simulink model "ALL_Test"  (R2021b)
settings: Solver=VariableStepAuto  StartTime=0.0  StopTime=0.1  RelTol=1e-3
undefined symbols (not defined in the file): ac, ma
libraries: fl_lib x142, nesl_utility x5, sdl_lib x1
settings Model: Creator=김웅지  LastModifiedBy=김웅지

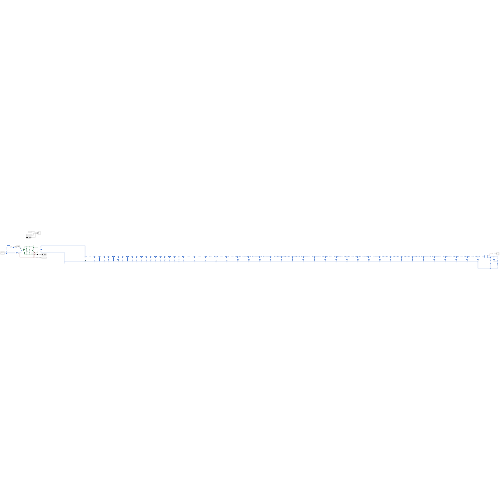
[thumbnail: Simulink's stored preview of the top-level diagram]
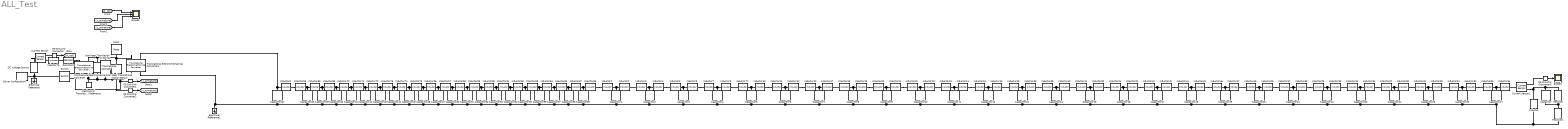
== system ALL_Test ==
  Capacitor : fl_lib/Electrical/Electrical Elements/Capacitor  c=ac.rad.Cm1 F  r=1e-15 Ohm  g=0 1/Ohm  i_specify=off  i_priority=None  i=0 A  i_nominal_specify=off  i_nominal_unit=A  i_nominal_value=1  v_specify=off  v_priority=None  v=0 V  v_nominal_specify=off  v_nominal_unit=V  v_nominal_value=1  vc_specify=off  vc_priority=High  vc=0 V  vc_nominal_specify=off  vc_nominal_unit=V  vc_nominal_value=1
  Capacitor1 : fl_lib/Electrical/Electrical Elements/Capacitor  c=ac.ho.C(1) F  r=1e-15 Ohm  g=0 1/Ohm  i_specify=off  i_priority=None  i=0 A  i_nominal_specify=off  i_nominal_unit=A  i_nominal_value=1  v_specify=off  v_priority=None  v=0 V  v_nominal_specify=off  v_nominal_unit=V  v_nominal_value=1  vc_specify=off  vc_priority=High  vc=0 V  vc_nominal_specify=off  vc_nominal_unit=V  vc_nominal_value=1
  Capacitor10 : fl_lib/Electrical/Electrical Elements/Capacitor  c=ac.ho.C(10) F  r=1e-15 Ohm  g=0 1/Ohm  i_specify=off  i_priority=None  i=0 A  i_nominal_specify=off  i_nominal_unit=A  i_nominal_value=1  v_specify=off  v_priority=None  v=0 V  v_nominal_specify=off  v_nominal_unit=V  v_nominal_value=1  vc_specify=off  vc_priority=High  vc=0 V  vc_nominal_specify=off  vc_nominal_unit=V  vc_nominal_value=1
  Capacitor11 : fl_lib/Electrical/Electrical Elements/Capacitor  c=ac.ho.C(11) F  r=1e-15 Ohm  g=0 1/Ohm  i_specify=off  i_priority=None  i=0 A  i_nominal_specify=off  i_nominal_unit=A  i_nominal_value=1  v_specify=off  v_priority=None  v=0 V  v_nominal_specify=off  v_nominal_unit=V  v_nominal_value=1  vc_specify=off  vc_priority=High  vc=0 V  vc_nominal_specify=off  vc_nominal_unit=V  vc_nominal_value=1
  Capacitor12 : fl_lib/Electrical/Electrical Elements/Capacitor  c=ac.ho.C(12) F  r=1e-15 Ohm  g=0 1/Ohm  i_specify=off  i_priority=None  i=0 A  i_nominal_specify=off  i_nominal_unit=A  i_nominal_value=1  v_specify=off  v_priority=None  v=0 V  v_nominal_specify=off  v_nominal_unit=V  v_nominal_value=1  vc_specify=off  vc_priority=High  vc=0 V  vc_nominal_specify=off  vc_nominal_unit=V  vc_nominal_value=1
  Capacitor13 : fl_lib/Electrical/Electrical Elements/Capacitor  c=ac.ho.C(13) F  r=1e-15 Ohm  g=0 1/Ohm  i_specify=off  i_priority=None  i=0 A  i_nominal_specify=off  i_nominal_unit=A  i_nominal_value=1  v_specify=off  v_priority=None  v=0 V  v_nominal_specify=off  v_nominal_unit=V  v_nominal_value=1  vc_specify=off  vc_priority=High  vc=0 V  vc_nominal_specify=off  vc_nominal_unit=V  vc_nominal_value=1
  Capacitor14 : fl_lib/Electrical/Electrical Elements/Capacitor  c=ac.ho.C(14) F  r=1e-15 Ohm  g=0 1/Ohm  i_specify=off  i_priority=None  i=0 A  i_nominal_specify=off  i_nominal_unit=A  i_nominal_value=1  v_specify=off  v_priority=None  v=0 V  v_nominal_specify=off  v_nominal_unit=V  v_nominal_value=1  vc_specify=off  vc_priority=High  vc=0 V  vc_nominal_specify=off  vc_nominal_unit=V  vc_nominal_value=1
  Capacitor15 : fl_lib/Electrical/Electrical Elements/Capacitor  c=ac.ho.C(15) F  r=1e-15 Ohm  g=0 1/Ohm  i_specify=off  i_priority=None  i=0 A  i_nominal_specify=off  i_nominal_unit=A  i_nominal_value=1  v_specify=off  v_priority=None  v=0 V  v_nominal_specify=off  v_nominal_unit=V  v_nominal_value=1  vc_specify=off  vc_priority=High  vc=0 V  vc_nominal_specify=off  vc_nominal_unit=V  vc_nominal_value=1
  Capacitor16 : fl_lib/Electrical/Electrical Elements/Capacitor  c=ac.ho.C(16) F  r=1e-15 Ohm  g=0 1/Ohm  i_specify=off  i_priority=None  i=0 A  i_nominal_specify=off  i_nominal_unit=A  i_nominal_value=1  v_specify=off  v_priority=None  v=0 V  v_nominal_specify=off  v_nominal_unit=V  v_nominal_value=1  vc_specify=off  vc_priority=High  vc=0 V  vc_nominal_specify=off  vc_nominal_unit=V  vc_nominal_value=1
  Capacitor17 : fl_lib/Electrical/Electrical Elements/Capacitor  c=ac.ho.C(17) F  r=1e-15 Ohm  g=0 1/Ohm  i_specify=off  i_priority=None  i=0 A  i_nominal_specify=off  i_nominal_unit=A  i_nominal_value=1  v_specify=off  v_priority=None  v=0 V  v_nominal_specify=off  v_nominal_unit=V  v_nominal_value=1  vc_specify=off  vc_priority=High  vc=0 V  vc_nominal_specify=off  vc_nominal_unit=V  vc_nominal_value=1
  Capacitor18 : fl_lib/Electrical/Electrical Elements/Capacitor  c=ac.ho.C(18) F  r=1e-15 Ohm  g=0 1/Ohm  i_specify=off  i_priority=None  i=0 A  i_nominal_specify=off  i_nominal_unit=A  i_nominal_value=1  v_specify=off  v_priority=None  v=0 V  v_nominal_specify=off  v_nominal_unit=V  v_nominal_value=1  vc_specify=off  vc_priority=High  vc=0 V  vc_nominal_specify=off  vc_nominal_unit=V  vc_nominal_value=1
  Capacitor19 : fl_lib/Electrical/Electrical Elements/Capacitor  c=ac.ho.C(19) F  r=1e-15 Ohm  g=0 1/Ohm  i_specify=off  i_priority=None  i=0 A  i_nominal_specify=off  i_nominal_unit=A  i_nominal_value=1  v_specify=off  v_priority=None  v=0 V  v_nominal_specify=off  v_nominal_unit=V  v_nominal_value=1  vc_specify=off  vc_priority=High  vc=0 V  vc_nominal_specify=off  vc_nominal_unit=V  vc_nominal_value=1
  Capacitor2 : fl_lib/Electrical/Electrical Elements/Capacitor  c=ac.ho.C(2) F  r=1e-15 Ohm  g=0 1/Ohm  i_specify=off  i_priority=None  i=0 A  i_nominal_specify=off  i_nominal_unit=A  i_nominal_value=1  v_specify=off  v_priority=None  v=0 V  v_nominal_specify=off  v_nominal_unit=V  v_nominal_value=1  vc_specify=off  vc_priority=High  vc=0 V  vc_nominal_specify=off  vc_nominal_unit=V  vc_nominal_value=1
  Capacitor20 : fl_lib/Electrical/Electrical Elements/Capacitor  c=ac.ho.C(20) F  r=1e-15 Ohm  g=0 1/Ohm  i_specify=off  i_priority=None  i=0 A  i_nominal_specify=off  i_nominal_unit=A  i_nominal_value=1  v_specify=off  v_priority=None  v=0 V  v_nominal_specify=off  v_nominal_unit=V  v_nominal_value=1  vc_specify=off  vc_priority=High  vc=0 V  vc_nominal_specify=off  vc_nominal_unit=V  vc_nominal_value=1
  Capacitor21 : fl_lib/Electrical/Electrical Elements/Capacitor  c=ac.ho.C(21) F  r=1e-15 Ohm  g=0 1/Ohm  i_specify=off  i_priority=None  i=0 A  i_nominal_specify=off  i_nominal_unit=A  i_nominal_value=1  v_specify=off  v_priority=None  v=0 V  v_nominal_specify=off  v_nominal_unit=V  v_nominal_value=1  vc_specify=off  vc_priority=High  vc=0 V  vc_nominal_specify=off  vc_nominal_unit=V  vc_nominal_value=1
  Capacitor22 : fl_lib/Electrical/Electrical Elements/Capacitor  c=ac.ho.C(22) F  r=1e-15 Ohm  g=0 1/Ohm  i_specify=off  i_priority=None  i=0 A  i_nominal_specify=off  i_nominal_unit=A  i_nominal_value=1  v_specify=off  v_priority=None  v=0 V  v_nominal_specify=off  v_nominal_unit=V  v_nominal_value=1  vc_specify=off  vc_priority=High  vc=0 V  vc_nominal_specify=off  vc_nominal_unit=V  vc_nominal_value=1
  Capacitor23 : fl_lib/Electrical/Electrical Elements/Capacitor  c=ac.ho.C(23) F  r=1e-15 Ohm  g=0 1/Ohm  i_specify=off  i_priority=None  i=0 A  i_nominal_specify=off  i_nominal_unit=A  i_nominal_value=1  v_specify=off  v_priority=None  v=0 V  v_nominal_specify=off  v_nominal_unit=V  v_nominal_value=1  vc_specify=off  vc_priority=High  vc=0 V  vc_nominal_specify=off  vc_nominal_unit=V  vc_nominal_value=1
  Capacitor24 : fl_lib/Electrical/Electrical Elements/Capacitor  c=ac.ho.C(24) F  r=1e-15 Ohm  g=0 1/Ohm  i_specify=off  i_priority=None  i=0 A  i_nominal_specify=off  i_nominal_unit=A  i_nominal_value=1  v_specify=off  v_priority=None  v=0 V  v_nominal_specify=off  v_nominal_unit=V  v_nominal_value=1  vc_specify=off  vc_priority=High  vc=0 V  vc_nominal_specify=off  vc_nominal_unit=V  vc_nominal_value=1
  Capacitor25 : fl_lib/Electrical/Electrical Elements/Capacitor  c=ac.ho.C(25) F  r=1e-15 Ohm  g=0 1/Ohm  i_specify=off  i_priority=None  i=0 A  i_nominal_specify=off  i_nominal_unit=A  i_nominal_value=1  v_specify=off  v_priority=None  v=0 V  v_nominal_specify=off  v_nominal_unit=V  v_nominal_value=1  vc_specify=off  vc_priority=High  vc=0 V  vc_nominal_specify=off  vc_nominal_unit=V  vc_nominal_value=1
  Capacitor26 : fl_lib/Electrical/Electrical Elements/Capacitor  c=ac.ho.C(26) F  r=1e-15 Ohm  g=0 1/Ohm  i_specify=off  i_priority=None  i=0 A  i_nominal_specify=off  i_nominal_unit=A  i_nominal_value=1  v_specify=off  v_priority=None  v=0 V  v_nominal_specify=off  v_nominal_unit=V  v_nominal_value=1  vc_specify=off  vc_priority=High  vc=0 V  vc_nominal_specify=off  vc_nominal_unit=V  vc_nominal_value=1
  Capacitor27 : fl_lib/Electrical/Electrical Elements/Capacitor  c=ac.ho.C(27) F  r=1e-15 Ohm  g=0 1/Ohm  i_specify=off  i_priority=None  i=0 A  i_nominal_specify=off  i_nominal_unit=A  i_nominal_value=1  v_specify=off  v_priority=None  v=0 V  v_nominal_specify=off  v_nominal_unit=V  v_nominal_value=1  vc_specify=off  vc_priority=High  vc=0 V  vc_nominal_specify=off  vc_nominal_unit=V  vc_nominal_value=1
  Capacitor{28..47} (20 alike) : fl_lib/Electrical/Electrical Elements/Capacitor  c=ac.ps.C F  r=1e-15 Ohm  g=0 1/Ohm  i_specify=off  i_priority=None  i=0 A  i_nominal_specify=off  i_nominal_unit=A  i_nominal_value=1  v_specify=off  v_priority=None  v=0 V  v_nominal_specify=off  v_nominal_unit=V  v_nominal_value=1  vc_specify=off  vc_priority=High  vc=0 V  vc_nominal_specify=off  vc_nominal_unit=V  vc_nominal_value=1
  Capacitor3 : fl_lib/Electrical/Electrical Elements/Capacitor  c=ac.ho.C(3) F  r=1e-15 Ohm  g=0 1/Ohm  i_specify=off  i_priority=None  i=0 A  i_nominal_specify=off  i_nominal_unit=A  i_nominal_value=1  v_specify=off  v_priority=None  v=0 V  v_nominal_specify=off  v_nominal_unit=V  v_nominal_value=1  vc_specify=off  vc_priority=High  vc=0 V  vc_nominal_specify=off  vc_nominal_unit=V  vc_nominal_value=1
  Capacitor4 : fl_lib/Electrical/Electrical Elements/Capacitor  c=ac.ho.C(4) F  r=1e-15 Ohm  g=0 1/Ohm  i_specify=off  i_priority=None  i=0 A  i_nominal_specify=off  i_nominal_unit=A  i_nominal_value=1  v_specify=off  v_priority=None  v=0 V  v_nominal_specify=off  v_nominal_unit=V  v_nominal_value=1  vc_specify=off  vc_priority=High  vc=0 V  vc_nominal_specify=off  vc_nominal_unit=V  vc_nominal_value=1
  Capacitor48 : fl_lib/Electrical/Electrical Elements/Capacitor  c=ac.co.C F  r=1e-15 Ohm  g=0 1/Ohm  i_specify=off  i_priority=None  i=0 A  i_nominal_specify=off  i_nominal_unit=A  i_nominal_value=1  v_specify=off  v_priority=None  v=0 V  v_nominal_specify=off  v_nominal_unit=V  v_nominal_value=1  vc_specify=off  vc_priority=High  vc=0 V  vc_nominal_specify=off  vc_nominal_unit=V  vc_nominal_value=1
  Capacitor5 : fl_lib/Electrical/Electrical Elements/Capacitor  c=ac.ho.C(5) F  r=1e-15 Ohm  g=0 1/Ohm  i_specify=off  i_priority=None  i=0 A  i_nominal_specify=off  i_nominal_unit=A  i_nominal_value=1  v_specify=off  v_priority=None  v=0 V  v_nominal_specify=off  v_nominal_unit=V  v_nominal_value=1  vc_specify=off  vc_priority=High  vc=0 V  vc_nominal_specify=off  vc_nominal_unit=V  vc_nominal_value=1
  Capacitor6 : fl_lib/Electrical/Electrical Elements/Capacitor  c=ac.ho.C(6) F  r=1e-15 Ohm  g=0 1/Ohm  i_specify=off  i_priority=None  i=0 A  i_nominal_specify=off  i_nominal_unit=A  i_nominal_value=1  v_specify=off  v_priority=None  v=0 V  v_nominal_specify=off  v_nominal_unit=V  v_nominal_value=1  vc_specify=off  vc_priority=High  vc=0 V  vc_nominal_specify=off  vc_nominal_unit=V  vc_nominal_value=1
  Capacitor7 : fl_lib/Electrical/Electrical Elements/Capacitor  c=ac.ho.C(7) F  r=1e-15 Ohm  g=0 1/Ohm  i_specify=off  i_priority=None  i=0 A  i_nominal_specify=off  i_nominal_unit=A  i_nominal_value=1  v_specify=off  v_priority=None  v=0 V  v_nominal_specify=off  v_nominal_unit=V  v_nominal_value=1  vc_specify=off  vc_priority=High  vc=0 V  vc_nominal_specify=off  vc_nominal_unit=V  vc_nominal_value=1
  Capacitor8 : fl_lib/Electrical/Electrical Elements/Capacitor  c=ac.ho.C(8) F  r=1e-15 Ohm  g=0 1/Ohm  i_specify=off  i_priority=None  i=0 A  i_nominal_specify=off  i_nominal_unit=A  i_nominal_value=1  v_specify=off  v_priority=None  v=0 V  v_nominal_specify=off  v_nominal_unit=V  v_nominal_value=1  vc_specify=off  vc_priority=High  vc=0 V  vc_nominal_specify=off  vc_nominal_unit=V  vc_nominal_value=1
  Capacitor9 : fl_lib/Electrical/Electrical Elements/Capacitor  c=ac.ho.C(9) F  r=1e-15 Ohm  g=0 1/Ohm  i_specify=off  i_priority=None  i=0 A  i_nominal_specify=off  i_nominal_unit=A  i_nominal_value=1  v_specify=off  v_priority=None  v=0 V  v_nominal_specify=off  v_nominal_unit=V  v_nominal_value=1  vc_specify=off  vc_priority=High  vc=0 V  vc_nominal_specify=off  vc_nominal_unit=V  vc_nominal_value=1
  Current Sensor : fl_lib/Electrical/Electrical Sensors/Current Sensor
  Current Sensor1 : fl_lib/Electrical/Electrical Sensors/Current Sensor
  DC Voltage Source : fl_lib/Electrical/Electrical Sources/DC Voltage Source  v0=12 V
  Electrical Reference : fl_lib/Electrical/Electrical Elements/Electrical Reference
  Electrical Reference1 : fl_lib/Electrical/Electrical Elements/Electrical Reference
  Ideal Translational Motion Sensor : fl_lib/Mechanical/Mechanical Sensors/Ideal Translational Motion Sensor  offset=0 m
  Inductor : fl_lib/Electrical/Electrical Elements/Inductor  l=ac.rad.Mm1 H  r=0 Ohm  g=1e-15 1/Ohm  i_specify=off  i_priority=None  i=0 A  i_nominal_specify=off  i_nominal_unit=A  i_nominal_value=1  v_specify=off  v_priority=None  v=0 V  v_nominal_specify=off  v_nominal_unit=V  v_nominal_value=1  i_L_specify=off  i_L_priority=High  i_L=0 A  i_L_nominal_specify=off  i_L_nominal_unit=A  i_L_nominal_value=1
  Inductor1 : fl_lib/Electrical/Electrical Elements/Inductor  l=ac.ho.L(1) H  r=0 Ohm  g=1e-15 1/Ohm  i_specify=off  i_priority=None  i=0 A  i_nominal_specify=off  i_nominal_unit=A  i_nominal_value=1  v_specify=off  v_priority=None  v=0 V  v_nominal_specify=off  v_nominal_unit=V  v_nominal_value=1  i_L_specify=off  i_L_priority=High  i_L=0 A  i_L_nominal_specify=off  i_L_nominal_unit=A  i_L_nominal_value=1
  Inductor10 : fl_lib/Electrical/Electrical Elements/Inductor  l=ac.ho.L(5) H  r=0 Ohm  g=1e-15 1/Ohm  i_specify=off  i_priority=None  i=0 A  i_nominal_specify=off  i_nominal_unit=A  i_nominal_value=1  v_specify=off  v_priority=None  v=0 V  v_nominal_specify=off  v_nominal_unit=V  v_nominal_value=1  i_L_specify=off  i_L_priority=High  i_L=0 A  i_L_nominal_specify=off  i_L_nominal_unit=A  i_L_nominal_value=1
  Inductor11 : fl_lib/Electrical/Electrical Elements/Inductor  l=ac.ho.L(6) H  r=0 Ohm  g=1e-15 1/Ohm  i_specify=off  i_priority=None  i=0 A  i_nominal_specify=off  i_nominal_unit=A  i_nominal_value=1  v_specify=off  v_priority=None  v=0 V  v_nominal_specify=off  v_nominal_unit=V  v_nominal_value=1  i_L_specify=off  i_L_priority=High  i_L=0 A  i_L_nominal_specify=off  i_L_nominal_unit=A  i_L_nominal_value=1
  Inductor12 : fl_lib/Electrical/Electrical Elements/Inductor  l=ac.ho.L(6) H  r=0 Ohm  g=1e-15 1/Ohm  i_specify=off  i_priority=None  i=0 A  i_nominal_specify=off  i_nominal_unit=A  i_nominal_value=1  v_specify=off  v_priority=None  v=0 V  v_nominal_specify=off  v_nominal_unit=V  v_nominal_value=1  i_L_specify=off  i_L_priority=High  i_L=0 A  i_L_nominal_specify=off  i_L_nominal_unit=A  i_L_nominal_value=1
  Inductor13 : fl_lib/Electrical/Electrical Elements/Inductor  l=ac.ho.L(7) H  r=0 Ohm  g=1e-15 1/Ohm  i_specify=off  i_priority=None  i=0 A  i_nominal_specify=off  i_nominal_unit=A  i_nominal_value=1  v_specify=off  v_priority=None  v=0 V  v_nominal_specify=off  v_nominal_unit=V  v_nominal_value=1  i_L_specify=off  i_L_priority=High  i_L=0 A  i_L_nominal_specify=off  i_L_nominal_unit=A  i_L_nominal_value=1
  Inductor14 : fl_lib/Electrical/Electrical Elements/Inductor  l=ac.ho.L(11) H  r=0 Ohm  g=1e-15 1/Ohm  i_specify=off  i_priority=None  i=0 A  i_nominal_specify=off  i_nominal_unit=A  i_nominal_value=1  v_specify=off  v_priority=None  v=0 V  v_nominal_specify=off  v_nominal_unit=V  v_nominal_value=1  i_L_specify=off  i_L_priority=High  i_L=0 A  i_L_nominal_specify=off  i_L_nominal_unit=A  i_L_nominal_value=1
  Inductor15 : fl_lib/Electrical/Electrical Elements/Inductor  l=ac.ho.L(12) H  r=0 Ohm  g=1e-15 1/Ohm  i_specify=off  i_priority=None  i=0 A  i_nominal_specify=off  i_nominal_unit=A  i_nominal_value=1  v_specify=off  v_priority=None  v=0 V  v_nominal_specify=off  v_nominal_unit=V  v_nominal_value=1  i_L_specify=off  i_L_priority=High  i_L=0 A  i_L_nominal_specify=off  i_L_nominal_unit=A  i_L_nominal_value=1
  Inductor16 : fl_lib/Electrical/Electrical Elements/Inductor  l=ac.ho.L(12) H  r=0 Ohm  g=1e-15 1/Ohm  i_specify=off  i_priority=None  i=0 A  i_nominal_specify=off  i_nominal_unit=A  i_nominal_value=1  v_specify=off  v_priority=None  v=0 V  v_nominal_specify=off  v_nominal_unit=V  v_nominal_value=1  i_L_specify=off  i_L_priority=High  i_L=0 A  i_L_nominal_specify=off  i_L_nominal_unit=A  i_L_nominal_value=1
  Inductor17 : fl_lib/Electrical/Electrical Elements/Inductor  l=ac.ho.L(7) H  r=0 Ohm  g=1e-15 1/Ohm  i_specify=off  i_priority=None  i=0 A  i_nominal_specify=off  i_nominal_unit=A  i_nominal_value=1  v_specify=off  v_priority=None  v=0 V  v_nominal_specify=off  v_nominal_unit=V  v_nominal_value=1  i_L_specify=off  i_L_priority=High  i_L=0 A  i_L_nominal_specify=off  i_L_nominal_unit=A  i_L_nominal_value=1
  Inductor18 : fl_lib/Electrical/Electrical Elements/Inductor  l=ac.ho.L(8) H  r=0 Ohm  g=1e-15 1/Ohm  i_specify=off  i_priority=None  i=0 A  i_nominal_specify=off  i_nominal_unit=A  i_nominal_value=1  v_specify=off  v_priority=None  v=0 V  v_nominal_specify=off  v_nominal_unit=V  v_nominal_value=1  i_L_specify=off  i_L_priority=High  i_L=0 A  i_L_nominal_specify=off  i_L_nominal_unit=A  i_L_nominal_value=1
  Inductor19 : fl_lib/Electrical/Electrical Elements/Inductor  l=ac.ho.L(8) H  r=0 Ohm  g=1e-15 1/Ohm  i_specify=off  i_priority=None  i=0 A  i_nominal_specify=off  i_nominal_unit=A  i_nominal_value=1  v_specify=off  v_priority=None  v=0 V  v_nominal_specify=off  v_nominal_unit=V  v_nominal_value=1  i_L_specify=off  i_L_priority=High  i_L=0 A  i_L_nominal_specify=off  i_L_nominal_unit=A  i_L_nominal_value=1
  Inductor2 : fl_lib/Electrical/Electrical Elements/Inductor  l=ac.ho.L(1) H  r=0 Ohm  g=1e-15 1/Ohm  i_specify=off  i_priority=None  i=0 A  i_nominal_specify=off  i_nominal_unit=A  i_nominal_value=1  v_specify=off  v_priority=None  v=0 V  v_nominal_specify=off  v_nominal_unit=V  v_nominal_value=1  i_L_specify=off  i_L_priority=High  i_L=0 A  i_L_nominal_specify=off  i_L_nominal_unit=A  i_L_nominal_value=1
  Inductor20 : fl_lib/Electrical/Electrical Elements/Inductor  l=ac.ho.L(9) H  r=0 Ohm  g=1e-15 1/Ohm  i_specify=off  i_priority=None  i=0 A  i_nominal_specify=off  i_nominal_unit=A  i_nominal_value=1  v_specify=off  v_priority=None  v=0 V  v_nominal_specify=off  v_nominal_unit=V  v_nominal_value=1  i_L_specify=off  i_L_priority=High  i_L=0 A  i_L_nominal_specify=off  i_L_nominal_unit=A  i_L_nominal_value=1
  Inductor21 : fl_lib/Electrical/Electrical Elements/Inductor  l=ac.ho.L(9) H  r=0 Ohm  g=1e-15 1/Ohm  i_specify=off  i_priority=None  i=0 A  i_nominal_specify=off  i_nominal_unit=A  i_nominal_value=1  v_specify=off  v_priority=None  v=0 V  v_nominal_specify=off  v_nominal_unit=V  v_nominal_value=1  i_L_specify=off  i_L_priority=High  i_L=0 A  i_L_nominal_specify=off  i_L_nominal_unit=A  i_L_nominal_value=1
  Inductor22 : fl_lib/Electrical/Electrical Elements/Inductor  l=ac.ho.L(10) H  r=0 Ohm  g=1e-15 1/Ohm  i_specify=off  i_priority=None  i=0 A  i_nominal_specify=off  i_nominal_unit=A  i_nominal_value=1  v_specify=off  v_priority=None  v=0 V  v_nominal_specify=off  v_nominal_unit=V  v_nominal_value=1  i_L_specify=off  i_L_priority=High  i_L=0 A  i_L_nominal_specify=off  i_L_nominal_unit=A  i_L_nominal_value=1
  Inductor23 : fl_lib/Electrical/Electrical Elements/Inductor  l=ac.ho.L(10) H  r=0 Ohm  g=1e-15 1/Ohm  i_specify=off  i_priority=None  i=0 A  i_nominal_specify=off  i_nominal_unit=A  i_nominal_value=1  v_specify=off  v_priority=None  v=0 V  v_nominal_specify=off  v_nominal_unit=V  v_nominal_value=1  i_L_specify=off  i_L_priority=High  i_L=0 A  i_L_nominal_specify=off  i_L_nominal_unit=A  i_L_nominal_value=1
  Inductor24 : fl_lib/Electrical/Electrical Elements/Inductor  l=ac.ho.L(11) H  r=0 Ohm  g=1e-15 1/Ohm  i_specify=off  i_priority=None  i=0 A  i_nominal_specify=off  i_nominal_unit=A  i_nominal_value=1  v_specify=off  v_priority=None  v=0 V  v_nominal_specify=off  v_nominal_unit=V  v_nominal_value=1  i_L_specify=off  i_L_priority=High  i_L=0 A  i_L_nominal_specify=off  i_L_nominal_unit=A  i_L_nominal_value=1
  Inductor25 : fl_lib/Electrical/Electrical Elements/Inductor  l=ac.ho.L(13) H  r=0 Ohm  g=1e-15 1/Ohm  i_specify=off  i_priority=None  i=0 A  i_nominal_specify=off  i_nominal_unit=A  i_nominal_value=1  v_specify=off  v_priority=None  v=0 V  v_nominal_specify=off  v_nominal_unit=V  v_nominal_value=1  i_L_specify=off  i_L_priority=High  i_L=0 A  i_L_nominal_specify=off  i_L_nominal_unit=A  i_L_nominal_value=1
  Inductor26 : fl_lib/Electrical/Electrical Elements/Inductor  l=ac.ho.L(20) H  r=0 Ohm  g=1e-15 1/Ohm  i_specify=off  i_priority=None  i=0 A  i_nominal_specify=off  i_nominal_unit=A  i_nominal_value=1  v_specify=off  v_priority=None  v=0 V  v_nominal_specify=off  v_nominal_unit=V  v_nominal_value=1  i_L_specify=off  i_L_priority=High  i_L=0 A  i_L_nominal_specify=off  i_L_nominal_unit=A  i_L_nominal_value=1
  Inductor27 : fl_lib/Electrical/Electrical Elements/Inductor  l=ac.ho.L(21) H  r=0 Ohm  g=1e-15 1/Ohm  i_specify=off  i_priority=None  i=0 A  i_nominal_specify=off  i_nominal_unit=A  i_nominal_value=1  v_specify=off  v_priority=None  v=0 V  v_nominal_specify=off  v_nominal_unit=V  v_nominal_value=1  i_L_specify=off  i_L_priority=High  i_L=0 A  i_L_nominal_specify=off  i_L_nominal_unit=A  i_L_nominal_value=1
  Inductor28 : fl_lib/Electrical/Electrical Elements/Inductor  l=ac.ho.L(21) H  r=0 Ohm  g=1e-15 1/Ohm  i_specify=off  i_priority=None  i=0 A  i_nominal_specify=off  i_nominal_unit=A  i_nominal_value=1  v_specify=off  v_priority=None  v=0 V  v_nominal_specify=off  v_nominal_unit=V  v_nominal_value=1  i_L_specify=off  i_L_priority=High  i_L=0 A  i_L_nominal_specify=off  i_L_nominal_unit=A  i_L_nominal_value=1
  Inductor29 : fl_lib/Electrical/Electrical Elements/Inductor  l=ac.ho.L(22) H  r=0 Ohm  g=1e-15 1/Ohm  i_specify=off  i_priority=None  i=0 A  i_nominal_specify=off  i_nominal_unit=A  i_nominal_value=1  v_specify=off  v_priority=None  v=0 V  v_nominal_specify=off  v_nominal_unit=V  v_nominal_value=1  i_L_specify=off  i_L_priority=High  i_L=0 A  i_L_nominal_specify=off  i_L_nominal_unit=A  i_L_nominal_value=1
  Inductor3 : fl_lib/Electrical/Electrical Elements/Inductor  l=ac.ho.L(2) H  r=0 Ohm  g=1e-15 1/Ohm  i_specify=off  i_priority=None  i=0 A  i_nominal_specify=off  i_nominal_unit=A  i_nominal_value=1  v_specify=off  v_priority=None  v=0 V  v_nominal_specify=off  v_nominal_unit=V  v_nominal_value=1  i_L_specify=off  i_L_priority=High  i_L=0 A  i_L_nominal_specify=off  i_L_nominal_unit=A  i_L_nominal_value=1
  Inductor30 : fl_lib/Electrical/Electrical Elements/Inductor  l=ac.ho.L(15) H  r=0 Ohm  g=1e-15 1/Ohm  i_specify=off  i_priority=None  i=0 A  i_nominal_specify=off  i_nominal_unit=A  i_nominal_value=1  v_specify=off  v_priority=None  v=0 V  v_nominal_specify=off  v_nominal_unit=V  v_nominal_value=1  i_L_specify=off  i_L_priority=High  i_L=0 A  i_L_nominal_specify=off  i_L_nominal_unit=A  i_L_nominal_value=1
  Inductor31 : fl_lib/Electrical/Electrical Elements/Inductor  l=ac.ho.L(16) H  r=0 Ohm  g=1e-15 1/Ohm  i_specify=off  i_priority=None  i=0 A  i_nominal_specify=off  i_nominal_unit=A  i_nominal_value=1  v_specify=off  v_priority=None  v=0 V  v_nominal_specify=off  v_nominal_unit=V  v_nominal_value=1  i_L_specify=off  i_L_priority=High  i_L=0 A  i_L_nominal_specify=off  i_L_nominal_unit=A  i_L_nominal_value=1
  Inductor32 : fl_lib/Electrical/Electrical Elements/Inductor  l=ac.ho.L(16) H  r=0 Ohm  g=1e-15 1/Ohm  i_specify=off  i_priority=None  i=0 A  i_nominal_specify=off  i_nominal_unit=A  i_nominal_value=1  v_specify=off  v_priority=None  v=0 V  v_nominal_specify=off  v_nominal_unit=V  v_nominal_value=1  i_L_specify=off  i_L_priority=High  i_L=0 A  i_L_nominal_specify=off  i_L_nominal_unit=A  i_L_nominal_value=1
  Inductor33 : fl_lib/Electrical/Electrical Elements/Inductor  l=ac.ho.L(22) H  r=0 Ohm  g=1e-15 1/Ohm  i_specify=off  i_priority=None  i=0 A  i_nominal_specify=off  i_nominal_unit=A  i_nominal_value=1  v_specify=off  v_priority=None  v=0 V  v_nominal_specify=off  v_nominal_unit=V  v_nominal_value=1  i_L_specify=off  i_L_priority=High  i_L=0 A  i_L_nominal_specify=off  i_L_nominal_unit=A  i_L_nominal_value=1
  Inductor34 : fl_lib/Electrical/Electrical Elements/Inductor  l=ac.ho.L(23) H  r=0 Ohm  g=1e-15 1/Ohm  i_specify=off  i_priority=None  i=0 A  i_nominal_specify=off  i_nominal_unit=A  i_nominal_value=1  v_specify=off  v_priority=None  v=0 V  v_nominal_specify=off  v_nominal_unit=V  v_nominal_value=1  i_L_specify=off  i_L_priority=High  i_L=0 A  i_L_nominal_specify=off  i_L_nominal_unit=A  i_L_nominal_value=1
  Inductor35 : fl_lib/Electrical/Electrical Elements/Inductor  l=ac.ho.L(23) H  r=0 Ohm  g=1e-15 1/Ohm  i_specify=off  i_priority=None  i=0 A  i_nominal_specify=off  i_nominal_unit=A  i_nominal_value=1  v_specify=off  v_priority=None  v=0 V  v_nominal_specify=off  v_nominal_unit=V  v_nominal_value=1  i_L_specify=off  i_L_priority=High  i_L=0 A  i_L_nominal_specify=off  i_L_nominal_unit=A  i_L_nominal_value=1
  Inductor36 : fl_lib/Electrical/Electrical Elements/Inductor  l=ac.ho.L(13) H  r=0 Ohm  g=1e-15 1/Ohm  i_specify=off  i_priority=None  i=0 A  i_nominal_specify=off  i_nominal_unit=A  i_nominal_value=1  v_specify=off  v_priority=None  v=0 V  v_nominal_specify=off  v_nominal_unit=V  v_nominal_value=1  i_L_specify=off  i_L_priority=High  i_L=0 A  i_L_nominal_specify=off  i_L_nominal_unit=A  i_L_nominal_value=1
  Inductor37 : fl_lib/Electrical/Electrical Elements/Inductor  l=ac.ho.L(24) H  r=0 Ohm  g=1e-15 1/Ohm  i_specify=off  i_priority=None  i=0 A  i_nominal_specify=off  i_nominal_unit=A  i_nominal_value=1  v_specify=off  v_priority=None  v=0 V  v_nominal_specify=off  v_nominal_unit=V  v_nominal_value=1  i_L_specify=off  i_L_priority=High  i_L=0 A  i_L_nominal_specify=off  i_L_nominal_unit=A  i_L_nominal_value=1
  Inductor38 : fl_lib/Electrical/Electrical Elements/Inductor  l=ac.ho.L(24) H  r=0 Ohm  g=1e-15 1/Ohm  i_specify=off  i_priority=None  i=0 A  i_nominal_specify=off  i_nominal_unit=A  i_nominal_value=1  v_specify=off  v_priority=None  v=0 V  v_nominal_specify=off  v_nominal_unit=V  v_nominal_value=1  i_L_specify=off  i_L_priority=High  i_L=0 A  i_L_nominal_specify=off  i_L_nominal_unit=A  i_L_nominal_value=1
  Inductor39 : fl_lib/Electrical/Electrical Elements/Inductor  l=ac.ho.L(14) H  r=0 Ohm  g=1e-15 1/Ohm  i_specify=off  i_priority=None  i=0 A  i_nominal_specify=off  i_nominal_unit=A  i_nominal_value=1  v_specify=off  v_priority=None  v=0 V  v_nominal_specify=off  v_nominal_unit=V  v_nominal_value=1  i_L_specify=off  i_L_priority=High  i_L=0 A  i_L_nominal_specify=off  i_L_nominal_unit=A  i_L_nominal_value=1
  Inductor4 : fl_lib/Electrical/Electrical Elements/Inductor  l=ac.ho.L(2) H  r=0 Ohm  g=1e-15 1/Ohm  i_specify=off  i_priority=None  i=0 A  i_nominal_specify=off  i_nominal_unit=A  i_nominal_value=1  v_specify=off  v_priority=None  v=0 V  v_nominal_specify=off  v_nominal_unit=V  v_nominal_value=1  i_L_specify=off  i_L_priority=High  i_L=0 A  i_L_nominal_specify=off  i_L_nominal_unit=A  i_L_nominal_value=1
  Inductor40 : fl_lib/Electrical/Electrical Elements/Inductor  l=ac.ho.L(14) H  r=0 Ohm  g=1e-15 1/Ohm  i_specify=off  i_priority=None  i=0 A  i_nominal_specify=off  i_nominal_unit=A  i_nominal_value=1  v_specify=off  v_priority=None  v=0 V  v_nominal_specify=off  v_nominal_unit=V  v_nominal_value=1  i_L_specify=off  i_L_priority=High  i_L=0 A  i_L_nominal_specify=off  i_L_nominal_unit=A  i_L_nominal_value=1
  Inductor41 : fl_lib/Electrical/Electrical Elements/Inductor  l=ac.ho.L(15) H  r=0 Ohm  g=1e-15 1/Ohm  i_specify=off  i_priority=None  i=0 A  i_nominal_specify=off  i_nominal_unit=A  i_nominal_value=1  v_specify=off  v_priority=None  v=0 V  v_nominal_specify=off  v_nominal_unit=V  v_nominal_value=1  i_L_specify=off  i_L_priority=High  i_L=0 A  i_L_nominal_specify=off  i_L_nominal_unit=A  i_L_nominal_value=1
  Inductor42 : fl_lib/Electrical/Electrical Elements/Inductor  l=ac.ho.L(17) H  r=0 Ohm  g=1e-15 1/Ohm  i_specify=off  i_priority=None  i=0 A  i_nominal_specify=off  i_nominal_unit=A  i_nominal_value=1  v_specify=off  v_priority=None  v=0 V  v_nominal_specify=off  v_nominal_unit=V  v_nominal_value=1  i_L_specify=off  i_L_priority=High  i_L=0 A  i_L_nominal_specify=off  i_L_nominal_unit=A  i_L_nominal_value=1
  Inductor43 : fl_lib/Electrical/Electrical Elements/Inductor  l=ac.ho.L(17) H  r=0 Ohm  g=1e-15 1/Ohm  i_specify=off  i_priority=None  i=0 A  i_nominal_specify=off  i_nominal_unit=A  i_nominal_value=1  v_specify=off  v_priority=None  v=0 V  v_nominal_specify=off  v_nominal_unit=V  v_nominal_value=1  i_L_specify=off  i_L_priority=High  i_L=0 A  i_L_nominal_specify=off  i_L_nominal_unit=A  i_L_nominal_value=1
  Inductor44 : fl_lib/Electrical/Electrical Elements/Inductor  l=ac.ho.L(18) H  r=0 Ohm  g=1e-15 1/Ohm  i_specify=off  i_priority=None  i=0 A  i_nominal_specify=off  i_nominal_unit=A  i_nominal_value=1  v_specify=off  v_priority=None  v=0 V  v_nominal_specify=off  v_nominal_unit=V  v_nominal_value=1  i_L_specify=off  i_L_priority=High  i_L=0 A  i_L_nominal_specify=off  i_L_nominal_unit=A  i_L_nominal_value=1
  Inductor45 : fl_lib/Electrical/Electrical Elements/Inductor  l=ac.ho.L(18) H  r=0 Ohm  g=1e-15 1/Ohm  i_specify=off  i_priority=None  i=0 A  i_nominal_specify=off  i_nominal_unit=A  i_nominal_value=1  v_specify=off  v_priority=None  v=0 V  v_nominal_specify=off  v_nominal_unit=V  v_nominal_value=1  i_L_specify=off  i_L_priority=High  i_L=0 A  i_L_nominal_specify=off  i_L_nominal_unit=A  i_L_nominal_value=1
  Inductor46 : fl_lib/Electrical/Electrical Elements/Inductor  l=ac.ho.L(19) H  r=0 Ohm  g=1e-15 1/Ohm  i_specify=off  i_priority=None  i=0 A  i_nominal_specify=off  i_nominal_unit=A  i_nominal_value=1  v_specify=off  v_priority=None  v=0 V  v_nominal_specify=off  v_nominal_unit=V  v_nominal_value=1  i_L_specify=off  i_L_priority=High  i_L=0 A  i_L_nominal_specify=off  i_L_nominal_unit=A  i_L_nominal_value=1
  Inductor47 : fl_lib/Electrical/Electrical Elements/Inductor  l=ac.ho.L(19) H  r=0 Ohm  g=1e-15 1/Ohm  i_specify=off  i_priority=None  i=0 A  i_nominal_specify=off  i_nominal_unit=A  i_nominal_value=1  v_specify=off  v_priority=None  v=0 V  v_nominal_specify=off  v_nominal_unit=V  v_nominal_value=1  i_L_specify=off  i_L_priority=High  i_L=0 A  i_L_nominal_specify=off  i_L_nominal_unit=A  i_L_nominal_value=1
  Inductor48 : fl_lib/Electrical/Electrical Elements/Inductor  l=ac.ho.L(20) H  r=0 Ohm  g=1e-15 1/Ohm  i_specify=off  i_priority=None  i=0 A  i_nominal_specify=off  i_nominal_unit=A  i_nominal_value=1  v_specify=off  v_priority=None  v=0 V  v_nominal_specify=off  v_nominal_unit=V  v_nominal_value=1  i_L_specify=off  i_L_priority=High  i_L=0 A  i_L_nominal_specify=off  i_L_nominal_unit=A  i_L_nominal_value=1
  Inductor49 : fl_lib/Electrical/Electrical Elements/Inductor  l=ac.ho.L(25) H  r=0 Ohm  g=1e-15 1/Ohm  i_specify=off  i_priority=None  i=0 A  i_nominal_specify=off  i_nominal_unit=A  i_nominal_value=1  v_specify=off  v_priority=None  v=0 V  v_nominal_specify=off  v_nominal_unit=V  v_nominal_value=1  i_L_specify=off  i_L_priority=High  i_L=0 A  i_L_nominal_specify=off  i_L_nominal_unit=A  i_L_nominal_value=1
  Inductor5 : fl_lib/Electrical/Electrical Elements/Inductor  l=ac.ho.L(3) H  r=0 Ohm  g=1e-15 1/Ohm  i_specify=off  i_priority=None  i=0 A  i_nominal_specify=off  i_nominal_unit=A  i_nominal_value=1  v_specify=off  v_priority=None  v=0 V  v_nominal_specify=off  v_nominal_unit=V  v_nominal_value=1  i_L_specify=off  i_L_priority=High  i_L=0 A  i_L_nominal_specify=off  i_L_nominal_unit=A  i_L_nominal_value=1
  Inductor50 : fl_lib/Electrical/Electrical Elements/Inductor  l=ac.ho.L(25) H  r=0 Ohm  g=1e-15 1/Ohm  i_specify=off  i_priority=None  i=0 A  i_nominal_specify=off  i_nominal_unit=A  i_nominal_value=1  v_specify=off  v_priority=None  v=0 V  v_nominal_specify=off  v_nominal_unit=V  v_nominal_value=1  i_L_specify=off  i_L_priority=High  i_L=0 A  i_L_nominal_specify=off  i_L_nominal_unit=A  i_L_nominal_value=1
  Inductor51 : fl_lib/Electrical/Electrical Elements/Inductor  l=ac.ho.L(26) H  r=0 Ohm  g=1e-15 1/Ohm  i_specify=off  i_priority=None  i=0 A  i_nominal_specify=off  i_nominal_unit=A  i_nominal_value=1  v_specify=off  v_priority=None  v=0 V  v_nominal_specify=off  v_nominal_unit=V  v_nominal_value=1  i_L_specify=off  i_L_priority=High  i_L=0 A  i_L_nominal_specify=off  i_L_nominal_unit=A  i_L_nominal_value=1
  Inductor52 : fl_lib/Electrical/Electrical Elements/Inductor  l=ac.ho.L(26) H  r=0 Ohm  g=1e-15 1/Ohm  i_specify=off  i_priority=None  i=0 A  i_nominal_specify=off  i_nominal_unit=A  i_nominal_value=1  v_specify=off  v_priority=None  v=0 V  v_nominal_specify=off  v_nominal_unit=V  v_nominal_value=1  i_L_specify=off  i_L_priority=High  i_L=0 A  i_L_nominal_specify=off  i_L_nominal_unit=A  i_L_nominal_value=1
  Inductor53 : fl_lib/Electrical/Electrical Elements/Inductor  l=ac.ho.L(27) H  r=0 Ohm  g=1e-15 1/Ohm  i_specify=off  i_priority=None  i=0 A  i_nominal_specify=off  i_nominal_unit=A  i_nominal_value=1  v_specify=off  v_priority=None  v=0 V  v_nominal_specify=off  v_nominal_unit=V  v_nominal_value=1  i_L_specify=off  i_L_priority=High  i_L=0 A  i_L_nominal_specify=off  i_L_nominal_unit=A  i_L_nominal_value=1
  Inductor54 : fl_lib/Electrical/Electrical Elements/Inductor  l=ac.ho.L(27) H  r=0 Ohm  g=1e-15 1/Ohm  i_specify=off  i_priority=None  i=0 A  i_nominal_specify=off  i_nominal_unit=A  i_nominal_value=1  v_specify=off  v_priority=None  v=0 V  v_nominal_specify=off  v_nominal_unit=V  v_nominal_value=1  i_L_specify=off  i_L_priority=High  i_L=0 A  i_L_nominal_specify=off  i_L_nominal_unit=A  i_L_nominal_value=1
  Inductor55 : fl_lib/Electrical/Electrical Elements/Inductor  l=ac.ps.L/2 H  r=0 Ohm  g=1e-15 1/Ohm  i_specify=off  i_priority=None  i=0 A  i_nominal_specify=off  i_nominal_unit=A  i_nominal_value=1  v_specify=off  v_priority=None  v=0 V  v_nominal_specify=off  v_nominal_unit=V  v_nominal_value=1  i_L_specify=off  i_L_priority=High  i_L=0 A  i_L_nominal_specify=off  i_L_nominal_unit=A  i_L_nominal_value=1
  Inductor{56..67,69..75} (19 alike) : fl_lib/Electrical/Electrical Elements/Inductor  l=ac.ps.L H  r=0 Ohm  g=1e-15 1/Ohm  i_specify=off  i_priority=None  i=0 A  i_nominal_specify=off  i_nominal_unit=A  i_nominal_value=1  v_specify=off  v_priority=None  v=0 V  v_nominal_specify=off  v_nominal_unit=V  v_nominal_value=1  i_L_specify=off  i_L_priority=High  i_L=0 A  i_L_nominal_specify=off  i_L_nominal_unit=A  i_L_nominal_value=1
  Inductor6 : fl_lib/Electrical/Electrical Elements/Inductor  l=ac.ho.L(3) H  r=0 Ohm  g=1e-15 1/Ohm  i_specify=off  i_priority=None  i=0 A  i_nominal_specify=off  i_nominal_unit=A  i_nominal_value=1  v_specify=off  v_priority=None  v=0 V  v_nominal_specify=off  v_nominal_unit=V  v_nominal_value=1  i_L_specify=off  i_L_priority=High  i_L=0 A  i_L_nominal_specify=off  i_L_nominal_unit=A  i_L_nominal_value=1
  Inductor68 : fl_lib/Electrical/Electrical Elements/Inductor  l=ac.ps.L/2 H  r=0 Ohm  g=1e-15 1/Ohm  i_specify=off  i_priority=None  i=0 A  i_nominal_specify=off  i_nominal_unit=A  i_nominal_value=1  v_specify=off  v_priority=None  v=0 V  v_nominal_specify=off  v_nominal_unit=V  v_nominal_value=1  i_L_specify=off  i_L_priority=High  i_L=0 A  i_L_nominal_specify=off  i_L_nominal_unit=A  i_L_nominal_value=1
  Inductor7 : fl_lib/Electrical/Electrical Elements/Inductor  l=ac.ho.L(4) H  r=0 Ohm  g=1e-15 1/Ohm  i_specify=off  i_priority=None  i=0 A  i_nominal_specify=off  i_nominal_unit=A  i_nominal_value=1  v_specify=off  v_priority=None  v=0 V  v_nominal_specify=off  v_nominal_unit=V  v_nominal_value=1  i_L_specify=off  i_L_priority=High  i_L=0 A  i_L_nominal_specify=off  i_L_nominal_unit=A  i_L_nominal_value=1
  Inductor76 : fl_lib/Electrical/Electrical Elements/Inductor  l=2e-3 H  r=0 Ohm  g=1e-12 1/Ohm  i_specify=off  i_priority=None  i=0 A  i_nominal_specify=off  i_nominal_unit=A  i_nominal_value=1  v_specify=off  v_priority=None  v=0 V  v_nominal_specify=off  v_nominal_unit=V  v_nominal_value=1  i_L_specify=off  i_L_priority=High  i_L=0 A  i_L_nominal_specify=off  i_L_nominal_unit=A  i_L_nominal_value=1
  Inductor77 : fl_lib/Electrical/Electrical Elements/Inductor  l=ac.ho.L(5) H  r=0 Ohm  g=1e-15 1/Ohm  i_specify=off  i_priority=None  i=0 A  i_nominal_specify=off  i_nominal_unit=A  i_nominal_value=1  v_specify=off  v_priority=None  v=0 V  v_nominal_specify=off  v_nominal_unit=V  v_nominal_value=1  i_L_specify=off  i_L_priority=High  i_L=0 A  i_L_nominal_specify=off  i_L_nominal_unit=A  i_L_nominal_value=1
  Inductor8 : fl_lib/Electrical/Electrical Elements/Inductor  l=ac.co.L H  r=0 Ohm  g=1e-15 1/Ohm  i_specify=off  i_priority=None  i=0 A  i_nominal_specify=off  i_nominal_unit=A  i_nominal_value=1  v_specify=off  v_priority=None  v=0 V  v_nominal_specify=off  v_nominal_unit=V  v_nominal_value=1  i_L_specify=off  i_L_priority=High  i_L=0 A  i_L_nominal_specify=off  i_L_nominal_unit=A  i_L_nominal_value=1
  Inductor9 : fl_lib/Electrical/Electrical Elements/Inductor  l=ac.ho.L(4) H  r=0 Ohm  g=1e-15 1/Ohm  i_specify=off  i_priority=None  i=0 A  i_nominal_specify=off  i_nominal_unit=A  i_nominal_value=1  v_specify=off  v_priority=None  v=0 V  v_nominal_specify=off  v_nominal_unit=V  v_nominal_value=1  i_L_specify=off  i_L_priority=High  i_L=0 A  i_L_nominal_specify=off  i_L_nominal_unit=A  i_L_nominal_value=1
  Mass : fl_lib/Mechanical/Translational Elements/Mass  mass=28 g  num_ports=foundation.enum.numPorts2.one  v_specify=off  v_priority=High  v=0 m/s  v_nominal_specify=off  v_nominal_unit=m/s  v_nominal_value=1  f_specify=off  f_priority=None  f=0 N  f_nominal_specify=off  f_nominal_unit=N  f_nominal_value=1
  Mechanical Translational Reference : fl_lib/Mechanical/Translational Elements/Mechanical Translational Reference
  Nonlinear Translational Spring : sdl_lib/Couplings & Drives/Springs & Dampers/Nonlinear Translational Spring  parameterization=sdl.enum.polynomialTLU.polynomial  symmetry=sdl.enum.symmetry.symmetric  coefficient_vector=[146e3, 6e7, 1e11, 0, 0] N/m  tension_coefficient_vector=[145e3, 6e7, 1e11, 0, 0] N/m  compression_coefficient_vector=[145e3, 6e7, 1e11, 0, 0] N/m  deformation_vector=[-1, -.5, -.3, -.1, .1, .3, .5, 1] m  force_vector=[-1000, -400, -200, -50, 50, 200, 400, 1000] N  interp_method=simscape.enum.interpolation.linear  extrap_method=simscape.enum.extrapolation.linear  x_specify=off  x_priority=High  x=0 m  x_nominal_specify=off  x_nominal_unit=m  x_nominal_value=1
      settings: SourceProductBaseCode=LD  InternalSimscapePortConfiguration="{\"Bottom\":[],\"Left\":[{\"id\":\"R\",\"label\":\"R\",\"type\":\"foundation.mechanical.translational.translational\"}],\"Right\":[{\"id\":\"C\",\"label\":\"C\",\"type\":\"foundation.mechanical.translational.translational\"}],\"Top\":[]}"
  PS-Simulink Converter{,1..2,4} (4 alike) : nesl_utility/PS-Simulink Converter  PhysicalDomain=network_engine_domain  SubClassName=ps_output  LeftPortType=input  RightPortType=output  PseudoPeriodic=off  Frequencies=[]  Unit=inherit  AffineConversion=off
      settings: SourceProductBaseCode=PW,SS
  Resistor : fl_lib/Electrical/Electrical Elements/Resistor  R=ac.rad.Rm1 Ohm  i_specify=off  i_priority=None  i=0 A  i_nominal_specify=off  i_nominal_unit=A  i_nominal_value=1  v_specify=off  v_priority=None  v=0 V  v_nominal_specify=off  v_nominal_unit=V  v_nominal_value=1
  Resistor1 : fl_lib/Electrical/Electrical Elements/Resistor  R=ac.rad.Rm2 Ohm  i_specify=off  i_priority=None  i=0 A  i_nominal_specify=off  i_nominal_unit=A  i_nominal_value=1  v_specify=off  v_priority=None  v=0 V  v_nominal_specify=off  v_nominal_unit=V  v_nominal_value=1
  Resistor2 : fl_lib/Electrical/Electrical Elements/Resistor  R=0.55 Ohm  i_specify=off  i_priority=None  i=0 A  i_nominal_specify=off  i_nominal_unit=A  i_nominal_value=1  v_specify=off  v_priority=None  v=0 V  v_nominal_specify=off  v_nominal_unit=V  v_nominal_value=1
  Scope1 : Scope
  Scope2 : Scope  NumInputPorts=3
  Solver Configuration : nesl_utility/Solver Configuration  PhysicalDomain=network_engine_domain  SubClassName=solver  LeftPortType=input  RightPortType=generic  Tones=[]  Harmonics=[]  SimulateNoise=off  Profile=off  UseLocalSampling=off  EnableSwitchedLinearOptims=on  FrequencyDomain=off  UseCCode=off  RelTol=0.001  AbsTol=1e-06  MinStep=1e-09  ToWorkspace=off  RevertToSquareIcSolve=off  NumHomotopyIterations=100  PhasorMode=off  PhasorModeNumHarmonics=1  DoDC=off  ResidualTolerance=1e-09  UseLocalSolver=on  LocalSolverChoice=NE_BACKWARD_EULER_ADVANCER  LocalSolverSampleTime=1e-6  DoFixedCost=on  MaxNonlinIter=3  MaxModeIter=2  ComputeImpulses=off  ImpulseIterations=2  LinearAlgebra=auto  EquationFormulation=NE_TIME_EF  DelaysMemoryBudget=1024  AutomaticFiltering=on  FilteringTimeConstant=0.001  PartitionStorageMethod=AS_NEEDED  PartitionMemoryBudget=1024  PartitionMethod=ROBUST
      settings: SourceProductBaseCode=PW,SS
  Switch : fl_lib/Electrical/Electrical Elements/Switch  R_closed=1e-6 Ohm  G_open=1e-9 1/Ohm  Threshold=-200e-6  i_specify=off  i_priority=None  i=0 A  i_nominal_specify=off  i_nominal_unit=A  i_nominal_value=1  v_specify=off  v_priority=None  v=0 V  v_nominal_specify=off  v_nominal_unit=V  v_nominal_value=1
  Translational Electromechanical Converter : fl_lib/Electrical/Electrical Elements/Translational Electromechanical Converter  K=-1.8 N/A  i_specify=off  i_priority=None  i=0 A  i_nominal_specify=off  i_nominal_unit=A  i_nominal_value=1  v_specify=off  v_priority=None  v=0 V  v_nominal_specify=off  v_nominal_unit=V  v_nominal_value=1  f_specify=off  f_priority=None  f=0 N  f_nominal_specify=off  f_nominal_unit=N  f_nominal_value=1  u_specify=off  u_priority=None  u=0 m/s  u_nominal_specify=off  u_nominal_unit=m/s  u_nominal_value=1
      settings: SourceProductBaseCode=SS  InternalSimscapePortConfiguration="{\"Bottom\":[],\"Left\":[{\"id\":\"p\",\"label\":\"+\",\"type\":\"foundation.electrical.electrical\"},{\"id\":\"R\",\"label\":\"R\",\"type\":\"foundation.mechanical.translational.translational\"}],\"Right\":[{\"id\":\"n\",\"label\":\"-\",\"type\":\"foundation.electrical.electrical\"},{\"id\":\"C\",\"label\":\"C\",\"type\":\"foundation.mechanical.translational.translational\"}],\"Top\":[]}"
  Translational Electromechanical Converter1 : fl_lib/Electrical/Electrical Elements/Translational Electromechanical Converter  K=ma.co.DA N/A  i_specify=off  i_priority=None  i=0 A  i_nominal_specify=off  i_nominal_unit=A  i_nominal_value=1  v_specify=off  v_priority=None  v=0 V  v_nominal_specify=off  v_nominal_unit=V  v_nominal_value=1  f_specify=off  f_priority=None  f=0 N  f_nominal_specify=off  f_nominal_unit=N  f_nominal_value=1  u_specify=off  u_priority=None  u=0 m/s  u_nominal_specify=off  u_nominal_unit=m/s  u_nominal_value=1
      settings: SourceProductBaseCode=SS  InternalSimscapePortConfiguration="{\"Bottom\":[],\"Left\":[{\"id\":\"p\",\"label\":\"+\",\"type\":\"foundation.electrical.electrical\"},{\"id\":\"R\",\"label\":\"R\",\"type\":\"foundation.mechanical.translational.translational\"}],\"Right\":[{\"id\":\"n\",\"label\":\"-\",\"type\":\"foundation.electrical.electrical\"},{\"id\":\"C\",\"label\":\"C\",\"type\":\"foundation.mechanical.translational.translational\"}],\"Top\":[]}"
  Translational Damper : fl_lib/Mechanical/Translational Elements/Translational Damper  D=1 N/(m/s)  v_specify=off  v_priority=None  v=0 m/s  v_nominal_specify=off  v_nominal_unit=m/s  v_nominal_value=1  f_specify=off  f_priority=None  f=0 N  f_nominal_specify=off  f_nominal_unit=N  f_nominal_value=1
  wires:
  PS-Simulink Converter1/1 -> [x_armature]  "x"
  PS-Simulink Converter/1 -> [A_coil]  "i"
  PS-Simulink Converter2/1 -> [v_armature]  "v"
  [v_armature] -> Scope2/3
  [A_coil] -> Scope2/1
  [x_armature] -> Scope2/2
  PS-Simulink Converter4/1 -> Scope1/1
  connections:
  Mechanical Translational Reference/LConn1 -- Translational Electromechanical Converter1/RConn2 -- Ideal Translational Motion Sensor/RConn1 -- Nonlinear Translational Spring/RConn1 -- Translational Damper/RConn1 -- Translational Electromechanical Converter/RConn2
  Ideal Translational Motion Sensor/LConn1 -- Translational Damper/LConn1 -- Translational Electromechanical Converter/LConn2 -- Nonlinear Translational Spring/LConn1 -- Translational Electromechanical Converter1/LConn2 -- Mass/LConn1
  Electrical Reference/LConn1 -- DC Voltage Source/RConn1 -- Switch/LConn1 -- Solver Configuration/RConn1
  PS-Simulink Converter1/LConn1 -- Ideal Translational Motion Sensor/RConn3 -- Switch/RConn1
  Resistor2/LConn1 -- Inductor76/RConn1
  Switch/RConn2 -- Translational Electromechanical Converter/RConn1
  PS-Simulink Converter/LConn1 -- Current Sensor/RConn1
  Resistor2/RConn1 -- Translational Electromechanical Converter/LConn1
  Current Sensor/LConn1 -- DC Voltage Source/LConn1
  Ideal Translational Motion Sensor/RConn2 -- PS-Simulink Converter2/LConn1
  Current Sensor/RConn2 -- Inductor76/LConn1
  Inductor66/RConn1 -- Inductor69/LConn1 -- Capacitor29/LConn1
  Capacitor5/LConn1 -- Inductor10/LConn1 -- Inductor77/RConn1
  Inductor/LConn1 -- Current Sensor1/RConn2 -- Capacitor/LConn1 -- Resistor/LConn1
  Capacitor10/LConn1 -- Inductor23/LConn1 -- Inductor22/RConn1
  Capacitor16/LConn1 -- Inductor32/LConn1 -- Inductor31/RConn1
  Capacitor6/LConn1 -- Inductor12/LConn1 -- Inductor11/RConn1
  Resistor/RConn1 -- Capacitor/RConn1 -- Resistor1/LConn1
  Capacitor17/LConn1 -- Inductor43/LConn1 -- Inductor42/RConn1
  Capacitor8/LConn1 -- Inductor19/LConn1 -- Inductor18/RConn1
  Capacitor13/LConn1 -- Inductor36/LConn1 -- Inductor25/RConn1
  Inductor67/LConn1 -- Inductor65/RConn1 -- Capacitor38/LConn1
  Capacitor2/LConn1 -- Inductor4/LConn1 -- Inductor3/RConn1
  Inductor59/RConn1 -- Inductor60/LConn1 -- Capacitor32/LConn1
  Inductor63/LConn1 -- Inductor62/RConn1 -- Capacitor35/LConn1
  Capacitor1/LConn1 -- Inductor2/LConn1 -- Inductor1/RConn1
  Inductor67/RConn1 -- Inductor68/LConn1 -- Capacitor39/LConn1
  Capacitor22/LConn1 -- Inductor33/LConn1 -- Inductor29/RConn1
  Inductor57/RConn1 -- Inductor58/LConn1 -- Capacitor30/LConn1
  Capacitor27/LConn1 -- Inductor54/LConn1 -- Inductor53/RConn1
  Inductor75/LConn1 -- Inductor74/RConn1 -- Capacitor45/LConn1
  Inductor56/RConn1 -- Inductor57/LConn1 -- Capacitor47/LConn1
  Capacitor18/RConn1 -- Capacitor24/RConn1 -- Capacitor25/RConn1 -- Capacitor27/RConn1 -- Resistor1/RConn1 -- Inductor/RConn1 -- Capacitor26/RConn1 -- Capacitor23/RConn1 -- Capacitor22/RConn1 -- Capacitor21/RConn1 -- Capacitor20/RConn1 -- Capacitor19/RConn1 -- Capacitor38/RConn1 -- Capacitor37/RConn1 -- Capacitor36/RConn1 -- Capacitor35/RConn1 -- Capacitor34/RConn1 -- Capacitor33/RConn1 -- Capacitor32/RConn1 -- Capacitor31/RConn1 -- Capacitor30/RConn1 -- Capacitor47/RConn1 -- Capacitor46/RConn1 -- Capacitor45/RConn1 -- Capacitor44/RConn1 -- Capacitor43/RConn1 -- Capacitor42/RConn1 -- Capacitor41/RConn1 -- Capacitor40/RConn1 -- Capacitor29/RConn1 -- Translational Electromechanical Converter1/RConn1 -- Electrical Reference1/LConn1 -- Capacitor48/RConn1 -- Capacitor28/RConn1 -- Capacitor39/RConn1 -- Capacitor1/RConn1 -- Capacitor2/RConn1 -- Capacitor3/RConn1 -- Capacitor4/RConn1 -- Capacitor5/RConn1 -- Capacitor6/RConn1 -- Capacitor7/RConn1 -- Capacitor8/RConn1 -- Capacitor9/RConn1 -- Capacitor10/RConn1 -- Capacitor11/RConn1 -- Capacitor12/RConn1 -- Capacitor13/RConn1 -- Capacitor14/RConn1 -- Capacitor15/RConn1 -- Capacitor16/RConn1 -- Capacitor17/RConn1
  Inductor55/RConn1 -- Inductor66/LConn1 -- Capacitor28/LConn1
  Inductor62/LConn1 -- Inductor61/RConn1 -- Capacitor34/LConn1
  Capacitor24/LConn1 -- Inductor38/LConn1 -- Inductor37/RConn1
  Capacitor19/LConn1 -- Inductor47/LConn1 -- Inductor46/RConn1
  Inductor69/RConn1 -- Inductor70/LConn1 -- Capacitor40/LConn1
  Capacitor7/LConn1 -- Inductor17/LConn1 -- Inductor13/RConn1
  Inductor63/RConn1 -- Inductor64/LConn1 -- Capacitor36/LConn1
  Capacitor11/LConn1 -- Inductor14/LConn1 -- Inductor24/RConn1
  Capacitor26/LConn1 -- Inductor52/LConn1 -- Inductor51/RConn1
  Inductor61/LConn1 -- Inductor60/RConn1 -- Capacitor33/LConn1
  Capacitor3/LConn1 -- Inductor6/LConn1 -- Inductor5/RConn1
  Capacitor9/LConn1 -- Inductor21/LConn1 -- Inductor20/RConn1
  Capacitor18/LConn1 -- Inductor45/LConn1 -- Inductor44/RConn1
  Capacitor25/LConn1 -- Inductor50/LConn1 -- Inductor49/RConn1
  Capacitor21/LConn1 -- Inductor28/LConn1 -- Inductor27/RConn1
  Capacitor14/LConn1 -- Inductor40/LConn1 -- Inductor39/RConn1
  Capacitor15/LConn1 -- Inductor30/LConn1 -- Inductor41/RConn1
  Inductor74/LConn1 -- Inductor73/RConn1 -- Capacitor44/LConn1
  Inductor65/LConn1 -- Inductor64/RConn1 -- Capacitor37/LConn1
  Capacitor23/LConn1 -- Inductor35/LConn1 -- Inductor34/RConn1
  Inductor59/LConn1 -- Inductor58/RConn1 -- Capacitor31/LConn1
  Capacitor4/LConn1 -- Inductor9/LConn1 -- Inductor7/RConn1
  Capacitor48/LConn1 -- Translational Electromechanical Converter1/LConn1 -- Inductor8/LConn1
  Capacitor20/LConn1 -- Inductor26/LConn1 -- Inductor48/RConn1
  Capacitor12/LConn1 -- Inductor16/LConn1 -- Inductor15/RConn1
  Inductor71/RConn1 -- Inductor72/LConn1 -- Capacitor42/LConn1
  Inductor75/RConn1 -- Inductor56/LConn1 -- Capacitor46/LConn1
  Inductor73/LConn1 -- Inductor72/RConn1 -- Capacitor43/LConn1
  Inductor71/LConn1 -- Inductor70/RConn1 -- Capacitor41/LConn1
  Inductor10/RConn1 -- Inductor11/LConn1
  Inductor21/RConn1 -- Inductor22/LConn1
  Inductor43/RConn1 -- Inductor44/LConn1
  Inductor45/RConn1 -- Inductor46/LConn1
  Inductor14/RConn1 -- Inductor15/LConn1
  Inductor6/RConn1 -- Inductor7/LConn1
  Inductor26/RConn1 -- Inductor27/LConn1
  Inductor19/RConn1 -- Inductor20/LConn1
  Inductor48/LConn1 -- Inductor47/RConn1
  Inductor25/LConn1 -- Inductor16/RConn1
  Inductor32/RConn1 -- Inductor42/LConn1
  Inductor24/LConn1 -- Inductor23/RConn1
  Inductor39/LConn1 -- Inductor36/RConn1
  Inductor38/RConn1 -- Inductor49/LConn1
  Inductor51/LConn1 -- Inductor50/RConn1
  Inductor52/RConn1 -- Inductor53/LConn1
  Inductor4/RConn1 -- Inductor5/LConn1
  Inductor12/RConn1 -- Inductor13/LConn1
  Inductor30/RConn1 -- Inductor31/LConn1
  Inductor68/RConn1 -- Inductor1/LConn1
  Inductor34/LConn1 -- Inductor33/RConn1
  Inductor3/LConn1 -- Inductor2/RConn1
  Inductor77/LConn1 -- Inductor9/RConn1
  Inductor8/RConn1 -- Inductor55/LConn1
  Inductor41/LConn1 -- Inductor40/RConn1
  PS-Simulink Converter4/LConn1 -- Current Sensor1/RConn1
  Inductor18/LConn1 -- Inductor17/RConn1
  Current Sensor1/LConn1 -- Inductor54/RConn1
  Inductor28/RConn1 -- Inductor29/LConn1
  Inductor35/RConn1 -- Inductor37/LConn1
